simulink model "F550_CompareCA"  (R2024a)
settings: Solver=ode4  StartTime=0.0  StopTime=30  RelTol=1e-3
undefined symbols (not defined in the file or in its folder): r2d, SampleTime
libraries: slpidlib x21, simulink x9, simulink_extras x5
(part 1 of 3)
settings Model: Creator=UASG  LastModifiedBy=UASG

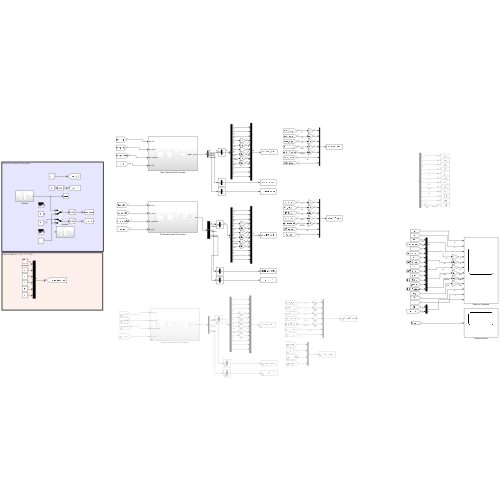
[thumbnail: Simulink's stored preview of the top-level diagram]
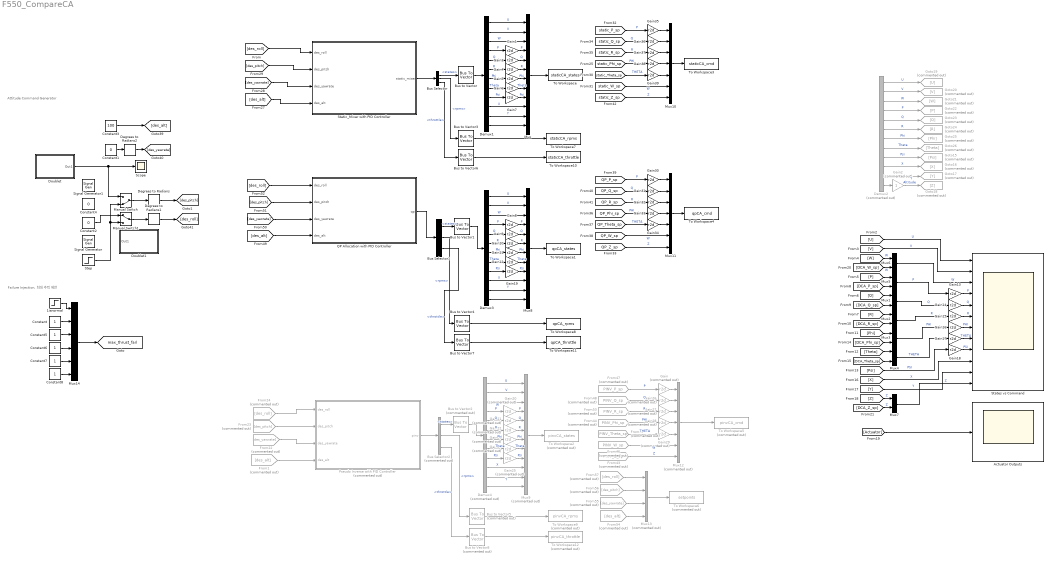
== system F550_CompareCA ==
  note: Failure Injection, 최대 추력 제한
  note: Attitude Command Generator
  1isnormal : Step  Time=10  Before=1  After=0.5
  Actuator Outputs : Scope
  Bus Selector : BusSelector  OutputSignals=states,rpms,throttle
  Bus Selector1 : BusSelector  OutputSignals=states,rpms,throttle
  Bus Selector2 : BusSelector  Commented=on  OutputSignals=states,rpms,throttle
  Bus to Vector{,1,3..4,6..7} (6 alike) : BusToVector
  Bus to Vector2 : BusToVector  Commented=on
  Bus to Vector5 : BusToVector  Commented=on
  Bus to Vector8 : BusToVector  Commented=on
  Constant{,5..8} (5 alike) : Constant
  Constant1 : Constant  Value=0
  Constant2 : Constant  Value=0
  Constant3 : Constant  Value=100
  Constant4 : Constant  Value=0
  Degrees to Radians : simulink_extras/Transformations/Degrees to Radians
  Degrees to Radians1 : simulink_extras/Transformations/Degrees to Radians
  Degrees to Radians2 : simulink_extras/Transformations/Degrees to Radians
  Demux1 : Demux  Outputs=12
  Demux2 : Demux  Commented=on  Outputs=12
  Demux3 : Demux  Outputs=12
  Demux4 : Demux  Commented=on  Outputs=12
  Doublet : Subsystem
  Doublet1 : Subsystem
  From1 : From  Commented=on  GotoTag=des_alt
  From22 : From  Commented=on  GotoTag=des_yawrate
  From23 : From  Commented=on  GotoTag=des_pitch
  From24 : From  Commented=on  GotoTag=des_roll
  From43 : From  Commented=on  GotoTag=PINV_Z_sp  TagVisibility=global
  From44 : From  Commented=on  GotoTag=PINV_Phi_sp  TagVisibility=global
  From45 : From  Commented=on  GotoTag=PINV_Theta_sp  TagVisibility=global
  From46 : From  Commented=on  GotoTag=PINV_W_sp  TagVisibility=global
  From47 : From  Commented=on  GotoTag=PINV_P_sp  TagVisibility=global
  From48 : From  Commented=on  GotoTag=PINV_Q_sp  TagVisibility=global
  From53 : From  Commented=on  GotoTag=PINV_R_sp  TagVisibility=global
  From54 : From  Commented=on  GotoTag=des_alt
  From55 : From  Commented=on  GotoTag=des_yawrate
  From56 : From  Commented=on  GotoTag=des_pitch
  From57 : From  Commented=on  GotoTag=des_roll
  Gain{,20..29} (11 alike) : Gain  Commented=on  Gain=r2d
  Gain{1,3..19,30..39} (28 alike) : Gain  Gain=r2d
  Gain2 : Gain  Commented=on
  Goto15 : Goto  Commented=on  GotoTag=Psi
  Goto16 : Goto  Commented=on  GotoTag=X
  Goto17 : Goto  Commented=on  GotoTag=Y
  Goto18 : Goto  Commented=on  GotoTag=Z
  Goto19 : Goto  Commented=on  GotoTag=U
  Goto20 : Goto  Commented=on  GotoTag=V
  Goto21 : Goto  Commented=on  GotoTag=W
  Goto22 : Goto  Commented=on  GotoTag=P
  Goto23 : Goto  Commented=on  GotoTag=Q
  Goto24 : Goto  Commented=on  GotoTag=R
  Goto25 : Goto  Commented=on  GotoTag=Phi
  Goto26 : Goto  Commented=on  GotoTag=Theta
  Manual Switch : ManualSwitch  CurrentSetting=0
  Manual Switch1 : ManualSwitch
  Mux : Mux  Inputs=12
  Mux{1..7} (7 alike) : Mux  Inputs=2
  Mux10 : Mux  Inputs=7
  Mux11 : Mux  Inputs=7
  Mux12 : Mux  Commented=on  Inputs=7
  Mux13 : Mux  Commented=on
  Mux14 : Mux  Inputs=6
  Mux8 : Mux  Inputs=12
  Mux9 : Mux  Commented=on  Inputs=12
  Pseudo Inverse with PID Controller : Subsystem  Commented=on
  QP Allocation with PID Controller : Subsystem
  Scope : Scope
  Signal Generator : SignalGenerator  Amplitude=4  Frequency=1/2
  Signal Generator1 : SignalGenerator  Amplitude=4  Frequency=1/2
  States vs Command : Scope  NumInputPorts=12
  Static_Mixer with PID Controller : Subsystem
  Step : Step  Time=5  After=10  SampleTime=0
  To Workspace : ToWorkspace  VariableName=staticCA_states  SampleTime=-1
  To Workspace1 : ToWorkspace  VariableName=qpCA_states  SampleTime=-1
  To Workspace10 : ToWorkspace  VariableName=staticCA_throttle  SampleTime=-1
      settings: Save2DSignal=2-D array (concatenate along first dimension)
  To Workspace11 : ToWorkspace  VariableName=qpCA_throttle  SampleTime=-1
      settings: Save2DSignal=2-D array (concatenate along first dimension)
  To Workspace12 : ToWorkspace  Commented=on  VariableName=pinvCA_throttle  SampleTime=-1
      settings: Save2DSignal=2-D array (concatenate along first dimension)
  To Workspace2 : ToWorkspace  Commented=on  VariableName=pinvCA_states  SampleTime=-1
  To Workspace3 : ToWorkspace  VariableName=staticCA_cmd  SampleTime=-1
  To Workspace4 : ToWorkspace  VariableName=qpCA_cmd  SampleTime=-1
  To Workspace5 : ToWorkspace  Commented=on  VariableName=pinvCA_cmd  SampleTime=-1
  To Workspace6 : ToWorkspace  Commented=on  VariableName=setpoints  SampleTime=-1
  To Workspace7 : ToWorkspace  VariableName=staticCA_rpms  SampleTime=-1
  To Workspace8 : ToWorkspace  VariableName=qpCA_rpms  SampleTime=-1
  To Workspace9 : ToWorkspace  Commented=on  VariableName=pinvCA_rpms  SampleTime=-1
  tag scope: max_thrust_fail=global
  wires:
  Constant2/1 -> Manual Switch1/1
  Degrees to Radians2/1 -> [des_yawrate]
  Degrees to Radians/1 -> [des_pitch]
  Degrees to Radians1/1 -> [des_roll]
  Manual Switch1/1 -> Degrees to Radians1/1
  Manual Switch/1 -> Degrees to Radians/1
  Constant1/1 -> Degrees to Radians2/1
  Constant3/1 -> [des_alt]
  Doublet/1(Out1) -> Manual Switch/1, Scope/1
  [DCA_Z_sp] -> Mux7/2  "Z"
  [Q] -> Mux1/1
  Gain18/1 -> States vs Command/9  "PSI"
  Gain15/1 -> States vs Command/6  "R"
  Gain17/1 -> States vs Command/8  "THETA"
  [DCA_W_sp] -> Mux6/2  "W"
  Gain16/1 -> States vs Command/7  "PHI"
  Gain13/1 -> States vs Command/4  "P"
  [DCA_Q_sp] -> Mux1/2
  [Phi] -> Mux3/1
  [DCA_Theta_sp] -> Mux4/2
  [Z] -> Mux7/1  "Z"
  [Actuator] -> Actuator Outputs/1
  [R] -> Mux2/1
  [Theta] -> Mux4/1
  [Psi] -> Gain18/1  "PSI"
  Mux4/1 -> Gain17/1  "THETA"
  Mux1/1 -> Gain14/1  "Q"
  Mux7/1 -> States vs Command/12  "Z"
  [X] -> States vs Command/10  "X"
  Mux3/1 -> Gain16/1  "PHI"
  Mux2/1 -> Gain15/1  "R"
  Mux6/1 -> States vs Command/3  "W"
  [W] -> Mux6/1  "W"
  Gain14/1 -> States vs Command/5  "Q"
  [DCA_Phi_sp] -> Mux3/2
  [V] -> States vs Command/2  "V"
  [U] -> States vs Command/1  "U"
  [P] -> Mux5/1
  [DCA_R_sp] -> Mux2/2
  Mux5/1 -> Gain13/1  "P"
  [Y] -> States vs Command/11  "Y"
  [DCA_P_sp] -> Mux5/2
  Gain2/1 -> Goto18/1  "Altitude"
  Demux2/12 -> Gain2/1
  Demux2/6 -> Goto24/1  "R"
  Demux2/9 -> Goto15/1  "Psi"
  Demux2/2 -> Goto20/1  "V"
  Demux2/5 -> Goto23/1  "Q"
  Demux2/4 -> Goto22/1  "P"
  Demux2/8 -> Goto26/1  "Theta"
  Demux2/3 -> Goto21/1  "W"
  Demux2/1 -> Goto19/1  "U"
  Demux2/11 -> Goto17/1  "Y"
  Demux2/10 -> Goto16/1  "X"
  Demux2/7 -> Goto25/1  "Phi"
  [des_roll] -> Static_Mixer with PID Controller/1(des_roll)
  [des_pitch] -> Static_Mixer with PID Controller/2(des_pitch)
  [des_yawrate] -> Static_Mixer with PID Controller/3(des_yawrate)
  [des_alt] -> Static_Mixer with PID Controller/4(des_alt)
  [des_roll] -> QP Allocation with PID Controller/1(des_roll)
  [des_pitch] -> QP Allocation with PID Controller/2(des_pitch)
  [des_yawrate] -> QP Allocation with PID Controller/3(des_yawrate)
  [des_alt] -> QP Allocation with PID Controller/4(des_alt)
  From24/1 -> Pseudo Inverse with PID Controller/1(des_roll)
  From23/1 -> Pseudo Inverse with PID Controller/2(des_pitch)
  From22/1 -> Pseudo Inverse with PID Controller/3(des_yawrate)
  From1/1 -> Pseudo Inverse with PID Controller/4(des_alt)
  Bus to Vector/1 -> Demux1/1
  Demux1/1 -> Mux/1  "U"
  Demux1/2 -> Mux/2  "V"
  Demux1/3 -> Mux/3  "W"
  Demux1/4 -> Gain1/1  "P"
  Gain1/1 -> Mux/4  "P"
  Demux1/5 -> Gain3/1  "Q"
  Gain3/1 -> Mux/5  "Q"
  Demux1/6 -> Gain4/1  "R"
  Demux1/7 -> Gain5/1  "Phi"
  Demux1/8 -> Gain6/1  "Theta"
  Demux1/9 -> Gain7/1  "Psi"
  Demux1/10 -> Mux/10  "X"
  Demux1/11 -> Mux/11  "Y"
  Demux1/12 -> Mux/12
  Gain7/1 -> Mux/9  "Psi"
  Gain6/1 -> Mux/8  "Theta"
  Gain5/1 -> Mux/7  "Phi"
  Gain4/1 -> Mux/6  "R"
  Mux/1 -> To Workspace/1
  Bus to Vector1/1 -> Demux3/1
  Gain10/1 -> Mux8/6  "R"
  Gain19/1 -> Mux8/9  "Psi"
  Gain11/1 -> Mux8/7  "Phi"
  Gain12/1 -> Mux8/8  "Theta"
  Demux3/8 -> Gain12/1  "Theta"
  Demux3/10 -> Mux8/10  "X"
  Gain9/1 -> Mux8/5  "Q"
  Demux3/3 -> Mux8/3  "W"
  Gain8/1 -> Mux8/4  "P"
  Demux3/12 -> Mux8/12
  Demux3/2 -> Mux8/2  "V"
  Demux3/11 -> Mux8/11  "Y"
  Demux3/4 -> Gain8/1  "P"
  Demux3/9 -> Gain19/1  "Psi"
  Mux8/1 -> To Workspace1/1
  Demux3/5 -> Gain9/1  "Q"
  Demux3/7 -> Gain11/1  "Phi"
  Demux3/6 -> Gain10/1  "R"
  Demux3/1 -> Mux8/1  "U"
  Bus to Vector2/1 -> Demux4/1
  Gain22/1 -> Mux9/6  "R"
  Gain25/1 -> Mux9/9  "Psi"
  Gain23/1 -> Mux9/7  "Phi"
  Gain24/1 -> Mux9/8  "Theta"
  Demux4/8 -> Gain24/1  "Theta"
  Demux4/10 -> Mux9/10  "X"
  Gain21/1 -> Mux9/5  "Q"
  Demux4/3 -> Mux9/3  "W"
  Gain20/1 -> Mux9/4  "P"
  Demux4/12 -> Mux9/12
  Demux4/2 -> Mux9/2  "V"
  Demux4/11 -> Mux9/11  "Y"
  Demux4/4 -> Gain20/1  "P"
  Demux4/9 -> Gain25/1  "Psi"
  Mux9/1 -> To Workspace2/1
  Demux4/5 -> Gain21/1  "Q"
  Demux4/7 -> Gain23/1  "Phi"
  Demux4/6 -> Gain22/1  "R"
  Demux4/1 -> Mux9/1  "U"
  [static_P_sp] -> Gain35/1  "P"
  [static_Q_sp] -> Gain36/1  "Q"
  [static_R_sp] -> Gain37/1  "R"
  [static_Phi_sp] -> Gain38/1  "PHI"
  [static_Theta_sp] -> Gain39/1  "THETA"
  [static_W_sp] -> Mux10/6  "W"
  Mux10/1 -> To Workspace3/1
  [QP_P_sp] -> Gain30/1  "P"
  [QP_R_sp] -> Gain32/1  "R"
  [QP_Theta_sp] -> Gain34/1  "THETA"
  [QP_Phi_sp] -> Gain33/1  "PHI"
  Mux11/1 -> To Workspace4/1
  [QP_W_sp] -> Mux11/6  "W"
  [QP_Q_sp] -> Gain31/1  "Q"
  [static_Z_sp] -> Mux10/7  "Z"
  [QP_Z_sp] -> Mux11/7  "Z"
  From46/1 -> Mux12/6  "W"
  From47/1 -> Gain/1  "P"
  From44/1 -> Gain28/1  "PHI"
  From48/1 -> Gain26/1  "Q"
  From43/1 -> Mux12/7  "Z"
  From53/1 -> Gain27/1  "R"
  From45/1 -> Gain29/1  "THETA"
  From57/1 -> Mux13/1
  From56/1 -> Mux13/2
  From55/1 -> Mux13/3
  From54/1 -> Mux13/4
  Mux13/1 -> To Workspace6/1
  Mux12/1 -> To Workspace5/1
  Gain/1 -> Mux12/1
  Gain26/1 -> Mux12/2
  Gain27/1 -> Mux12/3
  Gain28/1 -> Mux12/4
  Gain29/1 -> Mux12/5
  Gain30/1 -> Mux11/1
  Gain31/1 -> Mux11/2
  Gain32/1 -> Mux11/3
  Gain33/1 -> Mux11/4
  Gain34/1 -> Mux11/5
  Gain35/1 -> Mux10/1
  Gain36/1 -> Mux10/2
  Gain37/1 -> Mux10/3
  Gain38/1 -> Mux10/4
  Gain39/1 -> Mux10/5
  Static_Mixer with PID Controller/1(static_mixer) -> Bus Selector/1
  Bus Selector/1 -> Bus to Vector/1  "<states>"
  Bus Selector/2 -> Bus to Vector3/1  "<rpms>"
  Bus to Vector3/1 -> To Workspace7/1
  QP Allocation with PID Controller/1(qp) -> Bus Selector1/1
  Bus Selector1/1 -> Bus to Vector1/1  "<states>"
  Bus Selector1/2 -> Bus to Vector4/1  "<rpms>"
  Bus to Vector4/1 -> To Workspace8/1
  Pseudo Inverse with PID Controller/1(pinv) -> Bus Selector2/1
  Bus Selector2/1 -> Bus to Vector2/1  "<states>"
  Bus Selector2/2 -> Bus to Vector5/1  "<rpms>"
  Bus to Vector5/1 -> To Workspace9/1
  Bus Selector/3 -> Bus to Vector6/1  "<throttle>"
  Bus to Vector6/1 -> To Workspace10/1
  Bus to Vector7/1 -> To Workspace11/1
  Bus to Vector8/1 -> To Workspace12/1
  Bus Selector1/3 -> Bus to Vector7/1  "<throttle>"
  Bus Selector2/3 -> Bus to Vector8/1  "<throttle>"
  Step/1 -> Manual Switch/2, Manual Switch1/2
  1isnormal/1 -> Mux14/1
  Constant/1 -> Mux14/2
  Constant5/1 -> Mux14/3
  Constant6/1 -> Mux14/4
  Constant7/1 -> Mux14/5
  Constant8/1 -> Mux14/6
  Mux14/1 -> [max_thrust_fail]

== system F550_CompareCA/Doublet ==
  Add : Sum  Inputs=+++
  Step : Step  Time=10  After=8  SampleTime=0
  Step1 : Step  Time=15  After=-16  SampleTime=0
  Step2 : Step  Time=20  After=8  SampleTime=0
  Out1 : Outport
  wires:
  Step/1 -> Add/1
  Step1/1 -> Add/2
  Add/1 -> Out1/1
  Step2/1 -> Add/3

== system F550_CompareCA/Doublet1 ==
  Add : Sum  Inputs=+++
  Step : Step  Time=10  After=10  SampleTime=0
  Step1 : Step  Time=15  After=-20  SampleTime=0
  Step2 : Step  Time=20  After=10  SampleTime=0
  Out1 : Outport
  wires:
  Step/1 -> Add/1
  Step1/1 -> Add/2
  Add/1 -> Out1/1
  Step2/1 -> Add/3

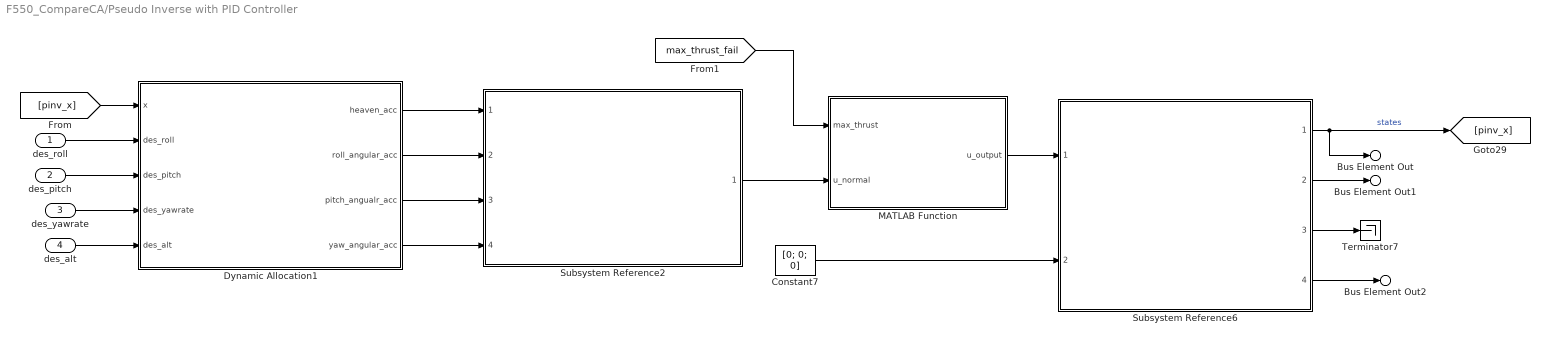
== system F550_CompareCA/Pseudo Inverse with PID Controller ==
  des_roll : Inport
  des_pitch : Inport  Port=2
  des_yawrate : Inport  Port=3
  des_alt : Inport  Port=4
  Constant7 : Constant  Value=[0; 0; 0]
  Dynamic Allocation1 : Subsystem
  MATLAB Function : MATLAB Function  TreatAsAtomicUnit=on
  Subsystem Reference2 : Subsystem  ReferencedSubsystem=F550_PseudoInv_ControlAllocation
  Subsystem Reference6 : Subsystem  ReferencedSubsystem=F550_Dynamics_sub_ver2023b
  Terminator7 : Terminator
  Bus Element Out : Outport  PortName=pinv  Element=states
  Bus Element Out1 : Outport  PortName=pinv  Element=rpms
  Bus Element Out2 : Outport  PortName=pinv  Element=throttle
  wires:
  Dynamic Allocation1/3(pitch_angualr_acc) -> Subsystem Reference2/3
  Dynamic Allocation1/1(heaven_acc) -> Subsystem Reference2/1
  Subsystem Reference6/1 -> Bus Element Out/1, [pinv_x]  "states"
  Dynamic Allocation1/4(yaw_angular_acc) -> Subsystem Reference2/4
  Subsystem Reference6/2 -> Bus Element Out1/1
  Dynamic Allocation1/2(roll_angular_acc) -> Subsystem Reference2/2
  Constant7/1 -> Subsystem Reference6/2
  des_yawrate/1 -> Dynamic Allocation1/4(des_yawrate)
  Subsystem Reference6/3 -> Terminator7/1
  des_roll/1 -> Dynamic Allocation1/2(des_roll)
  des_pitch/1 -> Dynamic Allocation1/3(des_pitch)
  des_alt/1 -> Dynamic Allocation1/5(des_alt)
  [pinv_x] -> Dynamic Allocation1/1(x)
  Subsystem Reference6/4 -> Bus Element Out2/1
  [max_thrust_fail] -> MATLAB Function/1(max_thrust)
  Subsystem Reference2/1 -> MATLAB Function/2(u_normal)
  MATLAB Function/1(u_output) -> Subsystem Reference6/1

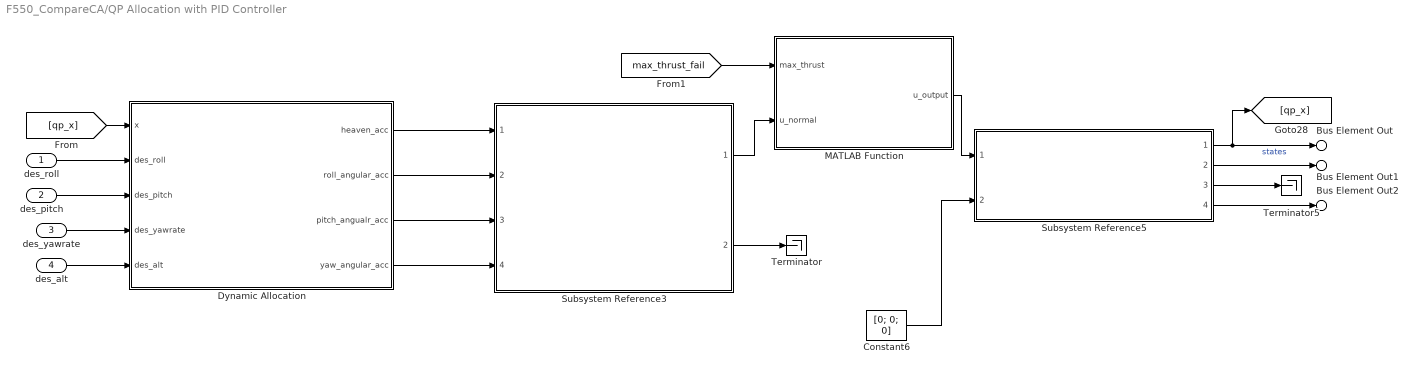
== system F550_CompareCA/QP Allocation with PID Controller ==
  des_roll : Inport
  des_pitch : Inport  Port=2
  des_yawrate : Inport  Port=3
  des_alt : Inport  Port=4
  Constant6 : Constant  Value=[0; 0; 0]
  Dynamic Allocation : Subsystem
  MATLAB Function : MATLAB Function  TreatAsAtomicUnit=on
  Subsystem Reference3 : Subsystem  ReferencedSubsystem=F550_Dynamic_CA
  Subsystem Reference5 : Subsystem  ReferencedSubsystem=F550_Dynamics_sub_ver2023b
  Terminator : Terminator
  Terminator5 : Terminator
  Bus Element Out : Outport  PortName=qp  Element=states
  Bus Element Out1 : Outport  PortName=qp  Element=rpms
  Bus Element Out2 : Outport  PortName=qp  Element=throttle
  wires:
  Subsystem Reference5/1 -> Bus Element Out/1, [qp_x]  "states"
  Dynamic Allocation/4(yaw_angular_acc) -> Subsystem Reference3/4
  Constant6/1 -> Subsystem Reference5/2
  Dynamic Allocation/3(pitch_angualr_acc) -> Subsystem Reference3/3
  Subsystem Reference5/3 -> Terminator5/1
  Dynamic Allocation/1(heaven_acc) -> Subsystem Reference3/1
  Dynamic Allocation/2(roll_angular_acc) -> Subsystem Reference3/2
  Subsystem Reference5/2 -> Bus Element Out1/1
  des_yawrate/1 -> Dynamic Allocation/4(des_yawrate)
  des_pitch/1 -> Dynamic Allocation/3(des_pitch)
  des_alt/1 -> Dynamic Allocation/5(des_alt)
  des_roll/1 -> Dynamic Allocation/2(des_roll)
  Subsystem Reference3/2 -> Terminator/1
  [qp_x] -> Dynamic Allocation/1(x)
  Subsystem Reference5/4 -> Bus Element Out2/1
  [max_thrust_fail] -> MATLAB Function/1(max_thrust)
  Subsystem Reference3/1 -> MATLAB Function/2(u_normal)
  MATLAB Function/1(u_output) -> Subsystem Reference5/1

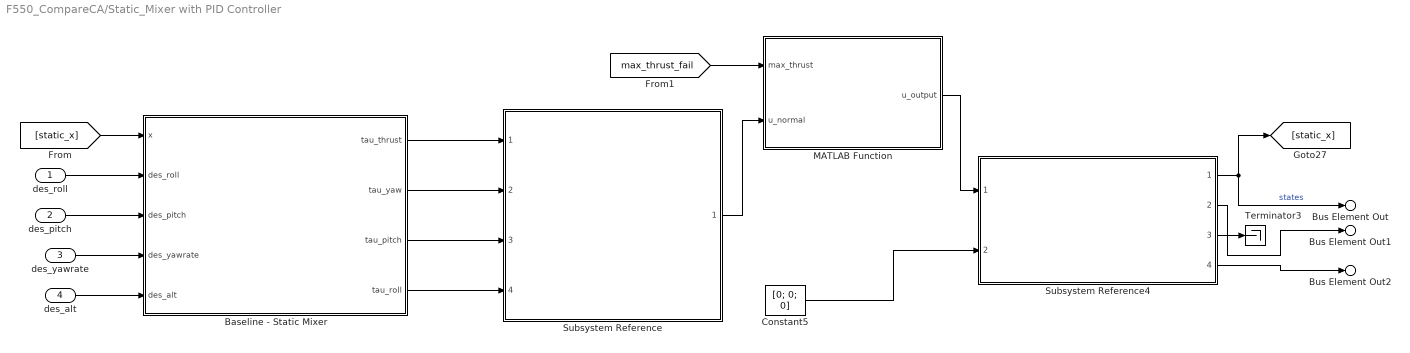
== system F550_CompareCA/Static_Mixer with PID Controller ==
  des_roll : Inport
  des_pitch : Inport  Port=2
  des_yawrate : Inport  Port=3
  des_alt : Inport  Port=4
  Baseline - Static Mixer : Subsystem
  Constant5 : Constant  Value=[0; 0; 0]
  MATLAB Function : MATLAB Function  TreatAsAtomicUnit=on
  Subsystem Reference : Subsystem  ReferencedSubsystem=F550_ControlAllocation_sub_ver2023b
  Subsystem Reference4 : Subsystem  ReferencedSubsystem=F550_Dynamics_sub_ver2023b
  Terminator3 : Terminator
  Bus Element Out : Outport  PortName=static_mixer  Element=states
  Bus Element Out1 : Outport  PortName=static_mixer  Element=rpms
  Bus Element Out2 : Outport  PortName=static_mixer  Element=throttle
  wires:
  Baseline - Static Mixer/4(tau_roll) -> Subsystem Reference/4
  Baseline - Static Mixer/2(tau_yaw) -> Subsystem Reference/2
  Baseline - Static Mixer/1(tau_thrust) -> Subsystem Reference/1
  Subsystem Reference4/1 -> Bus Element Out/1, [static_x]  "states"
  Baseline - Static Mixer/3(tau_pitch) -> Subsystem Reference/3
  Subsystem Reference4/3 -> Terminator3/1
  des_yawrate/1 -> Baseline - Static Mixer/4(des_yawrate)
  Constant5/1 -> Subsystem Reference4/2
  Subsystem Reference4/2 -> Bus Element Out1/1
  des_pitch/1 -> Baseline - Static Mixer/3(des_pitch)
  des_alt/1 -> Baseline - Static Mixer/5(des_alt)
  des_roll/1 -> Baseline - Static Mixer/2(des_roll)
  [static_x] -> Baseline - Static Mixer/1(x)
  Subsystem Reference4/4 -> Bus Element Out2/1
  Subsystem Reference/1 -> MATLAB Function/2(u_normal)
  MATLAB Function/1(u_output) -> Subsystem Reference4/1
  [max_thrust_fail] -> MATLAB Function/1(max_thrust)

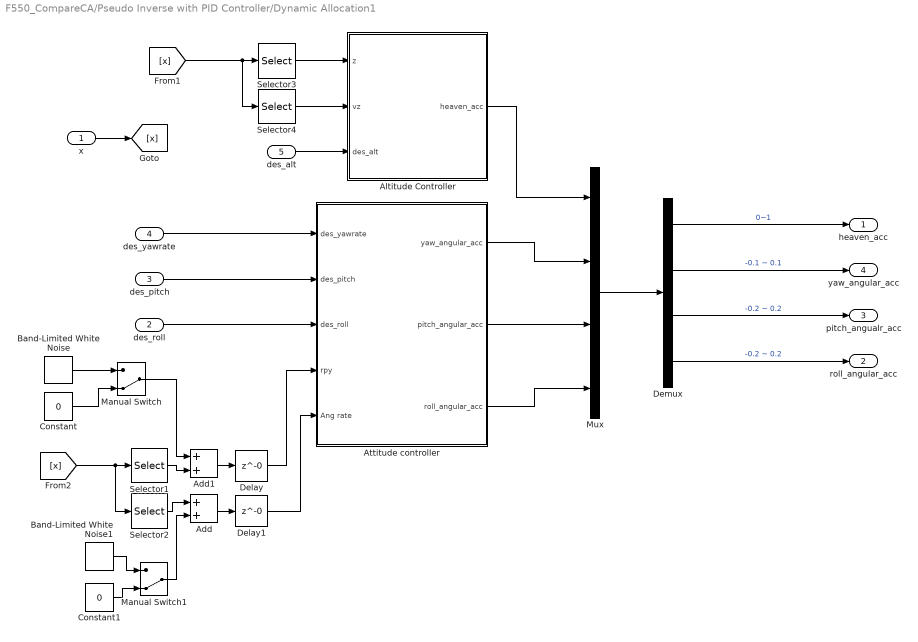
== system F550_CompareCA/Pseudo Inverse with PID Controller/Dynamic Allocation1 ==
  x : Inport
  des_roll : Inport  Port=2
  des_pitch : Inport  Port=3
  des_yawrate : Inport  Port=4
  des_alt : Inport  Port=5
  Add : Sum
  Add1 : Sum
  Altitude Controller : Subsystem
  Attitude controller : Subsystem
  Band-Limited White Noise : simulink/Sources/Band-Limited White Noise  Cov=[1e-5]  Ts=SampleTime  seed=[23341]
  Band-Limited White Noise1 : simulink/Sources/Band-Limited White Noise  Cov=[1e-6]  Ts=SampleTime  seed=[23341]
  Constant : Constant  Value=0
  Constant1 : Constant  Value=0
  Delay : Delay  DelayLength=0
  Delay1 : Delay  DelayLength=0
  Demux : Demux
  Manual Switch : ManualSwitch  CurrentSetting=0
  Manual Switch1 : ManualSwitch  CurrentSetting=0
  Mux : Mux
  Selector1 : Selector  InputPortWidth=12  IndexOptions=Index vector (dialog)  Indices=[7 8 9]  OutputSizes=1
  Selector2 : Selector  InputPortWidth=12  IndexOptions=Index vector (dialog)  Indices=[4 5 6]  OutputSizes=1
  Selector3 : Selector  InputPortWidth=12  IndexOptions=Index vector (dialog)  Indices=[12]  OutputSizes=1
  Selector4 : Selector  InputPortWidth=12  IndexOptions=Index vector (dialog)  Indices=[3]  OutputSizes=1
  heaven_acc : Outport
  roll_angular_acc : Outport  Port=2
  pitch_angualr_acc : Outport  Port=3
  yaw_angular_acc : Outport  Port=4
  wires:
  Add1/1 -> Delay/1
  Add/1 -> Delay1/1
  Selector2/1 -> Add/1
  Attitude controller/2(pitch_angular_acc) -> Mux/3
  Selector3/1 -> Altitude Controller/1(z)
  Selector4/1 -> Altitude Controller/2(vz)
  Attitude controller/3(roll_angular_acc) -> Mux/4
  Attitude controller/1(yaw_angular_acc) -> Mux/2
  Altitude Controller/1(heaven_acc) -> Mux/1
  Demux/2 -> yaw_angular_acc/1  "-0.1 ~ 0.1"
  Mux/1 -> Demux/1
  Demux/1 -> heaven_acc/1  "0~1"
  Demux/3 -> pitch_angualr_acc/1  "-0.2 ~ 0.2"
  Demux/4 -> roll_angular_acc/1  "-0.2 ~ 0.2"
  Delay/1 -> Attitude controller/4(rpy)
  [x] -> Selector4/1, Selector3/1
  Delay1/1 -> Attitude controller/5(Ang rate)
  [x] -> Selector2/1, Selector1/1
  x/1 -> [x]
  des_roll/1 -> Attitude controller/3(des_roll)
  des_pitch/1 -> Attitude controller/2(des_pitch)
  des_yawrate/1 -> Attitude controller/1(des_yawrate)
  des_alt/1 -> Altitude Controller/3(des_alt)
  Band-Limited White Noise/1 -> Manual Switch/1
  Selector1/1 -> Add1/2
  Manual Switch/1 -> Add1/1
  Constant/1 -> Manual Switch/2
  Band-Limited White Noise1/1 -> Manual Switch1/1
  Constant1/1 -> Manual Switch1/2
  Manual Switch1/1 -> Add/2

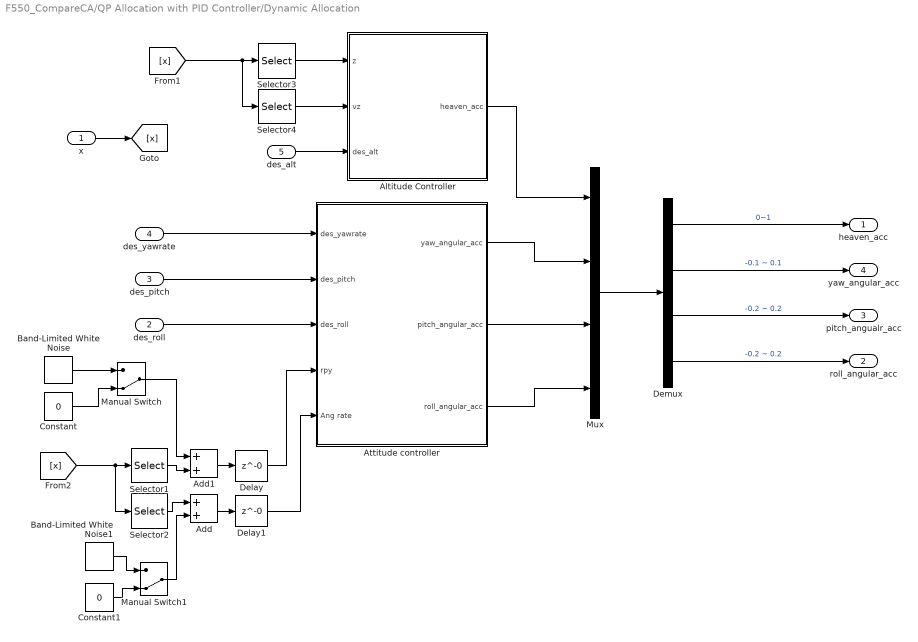
== system F550_CompareCA/QP Allocation with PID Controller/Dynamic Allocation ==
  x : Inport
  des_roll : Inport  Port=2
  des_pitch : Inport  Port=3
  des_yawrate : Inport  Port=4
  des_alt : Inport  Port=5
  Add : Sum
  Add1 : Sum
  Altitude Controller : Subsystem
  Attitude controller : Subsystem
  Band-Limited White Noise : simulink/Sources/Band-Limited White Noise  Cov=[1e-5]  Ts=SampleTime  seed=[23341]
  Band-Limited White Noise1 : simulink/Sources/Band-Limited White Noise  Cov=[1e-6]  Ts=SampleTime  seed=[23341]
  Constant : Constant  Value=0
  Constant1 : Constant  Value=0
  Delay : Delay  DelayLength=0
  Delay1 : Delay  DelayLength=0
  Demux : Demux
  Manual Switch : ManualSwitch  CurrentSetting=0
  Manual Switch1 : ManualSwitch  CurrentSetting=0
  Mux : Mux
  Selector1 : Selector  InputPortWidth=12  IndexOptions=Index vector (dialog)  Indices=[7 8 9]  OutputSizes=1
  Selector2 : Selector  InputPortWidth=12  IndexOptions=Index vector (dialog)  Indices=[4 5 6]  OutputSizes=1
  Selector3 : Selector  InputPortWidth=12  IndexOptions=Index vector (dialog)  Indices=[12]  OutputSizes=1
  Selector4 : Selector  InputPortWidth=12  IndexOptions=Index vector (dialog)  Indices=[3]  OutputSizes=1
  heaven_acc : Outport
  roll_angular_acc : Outport  Port=2
  pitch_angualr_acc : Outport  Port=3
  yaw_angular_acc : Outport  Port=4
  wires:
  Add1/1 -> Delay/1
  Add/1 -> Delay1/1
  Selector2/1 -> Add/1
  Attitude controller/2(pitch_angular_acc) -> Mux/3
  Selector3/1 -> Altitude Controller/1(z)
  Selector4/1 -> Altitude Controller/2(vz)
  Attitude controller/3(roll_angular_acc) -> Mux/4
  Attitude controller/1(yaw_angular_acc) -> Mux/2
  Altitude Controller/1(heaven_acc) -> Mux/1
  Demux/2 -> yaw_angular_acc/1  "-0.1 ~ 0.1"
  Mux/1 -> Demux/1
  Demux/1 -> heaven_acc/1  "0~1"
  Demux/3 -> pitch_angualr_acc/1  "-0.2 ~ 0.2"
  Demux/4 -> roll_angular_acc/1  "-0.2 ~ 0.2"
  Delay/1 -> Attitude controller/4(rpy)
  [x] -> Selector4/1, Selector3/1
  Delay1/1 -> Attitude controller/5(Ang rate)
  [x] -> Selector2/1, Selector1/1
  x/1 -> [x]
  des_roll/1 -> Attitude controller/3(des_roll)
  des_pitch/1 -> Attitude controller/2(des_pitch)
  des_yawrate/1 -> Attitude controller/1(des_yawrate)
  des_alt/1 -> Altitude Controller/3(des_alt)
  Band-Limited White Noise/1 -> Manual Switch/1
  Selector1/1 -> Add1/2
  Manual Switch/1 -> Add1/1
  Constant/1 -> Manual Switch/2
  Band-Limited White Noise1/1 -> Manual Switch1/1
  Constant1/1 -> Manual Switch1/2
  Manual Switch1/1 -> Add/2

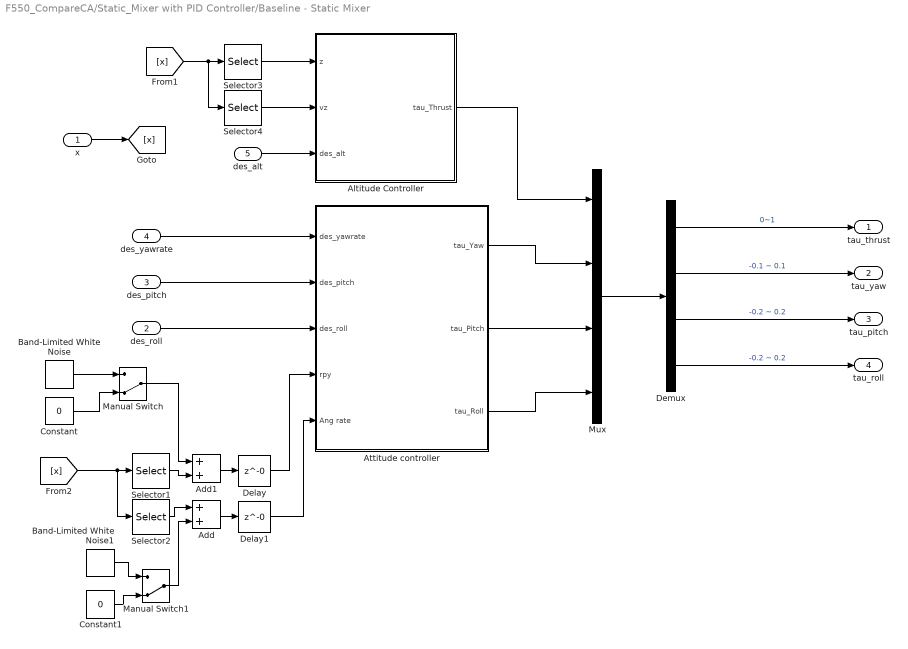
== system F550_CompareCA/Static_Mixer with PID Controller/Baseline - Static Mixer ==
  x : Inport
  des_roll : Inport  Port=2
  des_pitch : Inport  Port=3
  des_yawrate : Inport  Port=4
  des_alt : Inport  Port=5
  Add : Sum
  Add1 : Sum
  Altitude Controller : Subsystem
  Attitude controller : Subsystem
  Band-Limited White Noise : simulink/Sources/Band-Limited White Noise  Cov=[1e-5]  Ts=SampleTime  seed=[23341]
  Band-Limited White Noise1 : simulink/Sources/Band-Limited White Noise  Cov=[1e-6]  Ts=SampleTime  seed=[23341]
  Constant : Constant  Value=0
  Constant1 : Constant  Value=0
  Delay : Delay  DelayLength=0
  Delay1 : Delay  DelayLength=0
  Demux : Demux
  Manual Switch : ManualSwitch  CurrentSetting=0
  Manual Switch1 : ManualSwitch  CurrentSetting=0
  Mux : Mux
  Selector1 : Selector  InputPortWidth=12  IndexOptions=Index vector (dialog)  Indices=[7 8 9]  OutputSizes=1
  Selector2 : Selector  InputPortWidth=12  IndexOptions=Index vector (dialog)  Indices=[4 5 6]  OutputSizes=1
  Selector3 : Selector  InputPortWidth=12  IndexOptions=Index vector (dialog)  Indices=[12]  OutputSizes=1
  Selector4 : Selector  InputPortWidth=12  IndexOptions=Index vector (dialog)  Indices=[3]  OutputSizes=1
  tau_thrust : Outport
  tau_yaw : Outport  Port=2
  tau_pitch : Outport  Port=3
  tau_roll : Outport  Port=4
  wires:
  Attitude controller/2(tau_Pitch) -> Mux/3
  Selector3/1 -> Altitude Controller/1(z)
  Selector4/1 -> Altitude Controller/2(vz)
  Attitude controller/3(tau_Roll) -> Mux/4
  Attitude controller/1(tau_Yaw) -> Mux/2
  Altitude Controller/1(tau_Thrust) -> Mux/1
  Demux/2 -> tau_yaw/1  "-0.1 ~ 0.1"
  Mux/1 -> Demux/1
  Demux/1 -> tau_thrust/1  "0~1"
  Demux/3 -> tau_pitch/1  "-0.2 ~ 0.2"
  Demux/4 -> tau_roll/1  "-0.2 ~ 0.2"
  [x] -> Selector4/1, Selector3/1
  x/1 -> [x]
  des_roll/1 -> Attitude controller/3(des_roll)
  des_pitch/1 -> Attitude controller/2(des_pitch)
  des_yawrate/1 -> Attitude controller/1(des_yawrate)
  des_alt/1 -> Altitude Controller/3(des_alt)
  Manual Switch/1 -> Add1/1
  Constant1/1 -> Manual Switch1/2
  Band-Limited White Noise1/1 -> Manual Switch1/1
  Band-Limited White Noise/1 -> Manual Switch/1
  Manual Switch1/1 -> Add/2
  Constant/1 -> Manual Switch/2
  Selector1/1 -> Add1/2
  Delay1/1 -> Attitude controller/5(Ang rate)
  [x] -> Selector2/1, Selector1/1
  Selector2/1 -> Add/1
  Delay/1 -> Attitude controller/4(rpy)
  Add1/1 -> Delay/1
  Add/1 -> Delay1/1

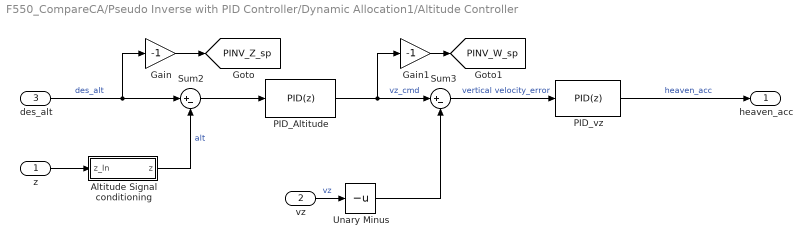
== system F550_CompareCA/Pseudo Inverse with PID Controller/Dynamic Allocation1/Altitude Controller ==
  z : Inport
  vz : Inport  Port=2
  des_alt : Inport  Port=3
  Altitude Signal conditioning : Subsystem
  Gain : Gain  Gain=-1
  Gain1 : Gain  Gain=-1
  PID_Altitude : slpidlib/PID Controller  Controller=PID  Form=Parallel  TimeDomain=Discrete-time  UseExternalTs=off  SampleTime=-1  IntegratorMethod=Backward Euler  FilterMethod=Forward Euler  ControllerParametersSource=internal  P=1  I=0  UseKiTs=off  D=0  UseExternalDerivativeSource=off  N=10  UseFilter=on  TunerSelectOption=Transfer Function Based (PID Tuner App)  InitialConditionSource=internal  InitialConditionForIntegrator=0  InitialConditionForFilter=0  DifferentiatorICPrevScaledInput=0  ExternalReset=none  TrackingMode=off  Kt=1  LimitOutput=on  SatLimitsSource=internal  UpperSaturationLimit=2  LowerSaturationLimit=-2  LinearizeAsGain=off  AntiWindupMode=clamping  Kb=1  LimitIntegrator=off  UpperIntegratorSaturationLimit=inf  LowerIntegratorSaturationLimit=-inf  POutMin=[]  POutMax=[]  IOutMin=[]  IOutMax=[]  DOutMin=[]  DOutMax=[]  NOutMin=[]  NOutMax=[]  SumOutMin=[]  SumOutMax=[]  SaturationOutMin=[]  SaturationOutMax=[]  PParamMin=[]  PParamMax=[]  IParamMin=[]  IParamMax=[]  DParamMin=[]  DParamMax=[]  NParamMin=[]  NParamMax=[]  KbParamMin=[]  KbParamMax=[]  KtParamMin=[]  KtParamMax=[]  KbOutMin=[]  KbOutMax=[]  KtOutMin=[]  KtOutMax=[]  IntegratorOutMin=[]  IntegratorOutMax=[]  FilterOutMin=[]  FilterOutMax=[]  SumI1OutMin=[]  SumI1OutMax=[]  SumI2OutMin=[]  SumI2OutMax=[]  SumI3OutMin=[]  SumI3OutMax=[]  SumI4OutMin=[]  SumI4OutMax=[]  SumDOutMin=[]  SumDOutMax=[]  DifferentiatorOutMin=[]  DifferentiatorOutMax=[]  FilterDiffOutCoefMin=[]  FilterDiffOutCoefMax=[]  ReciprocalOutMin=[]  ReciprocalOutMax=[]  SumDenOutMin=[]  SumDenOutMax=[]  SumNumOutMin=[]  SumNumOutMax=[]  DivideOutMin=[]  DivideOutMax=[]  UdiffTsProdOutMin=[]  UdiffTsProdOutMax=[]  NTsProdOutMin=[]  NTsProdOutMax=[]  UintegralTsProdOutMin=[]  UintegralTsProdOutMax=[]  UngainTsProdOutMin=[]  UngainTsProdOutMax=[]  ClampingZeroOutDataTypeStr=Inherit: Inherit via back propagation  ClampingZeroOutMin=[]  ClampingZeroOutMax=[]  FilterDenConstantOutDataTypeStr=Inherit: Inherit via back propagation  FilterDenConstantOutMin=[]  FilterDenConstantOutMax=[]  PCopyOutDataTypeStr=Inherit: Inherit via back propagation  PCopyOutMin=[]  PCopyOutMax=[]  NCopyOutDataTypeStr=Inherit: Inherit via back propagation  NCopyOutMin=[]  NCopyOutMax=[]  IntegratorContinuousStateAttributes=''  IntegratorStateMustResolveToSignalObject=off  IntegratorRTWStateStorageClass=Auto  FilterContinuousStateAttributes=''  FilterStateMustResolveToSignalObject=off  FilterRTWStateStorageClass=Auto  ParallelPVariant=InternalParameters  IdealPVariant=Disabled  IVariant=InternalParameters  DVariant=InternalParameters  IntegratorVariant=Discrete  SatVariant=Enabled  AWVariant=DiscClampingParallel  PCopyVariant=Disabled  TRVariant=Disabled  FdbkBlocksVariant=Feedback  IdealPFdbkVariant=Passthrough  SatFdbkVariant=Passthrough  DerivativeFilterVariant=ForwardEulerFilter  NVariant=InternalParameters  NCopyVariant=Disabled  FilterICVariant=InternalICsFilter  IntegratorICVariant=InternalICs  ExternalResetVariant=Disabled  TRSumVariant=Passthrough  SumFdbkVariant=Enabled  SumVariant=Sum_PID  TsampFilterVariant=InternalTs  TsampNgainVariant=Passthrough  TsampIntegralVariant=Disabled_SignalSpec  ExternalSaturationOutDataTypeStr=Inherit: Same as second input  DerivativeSourceVariant=ErrorSignal
  PID_vz : slpidlib/PID Controller  Controller=PID  Form=Parallel  TimeDomain=Discrete-time  UseExternalTs=off  SampleTime=-1  IntegratorMethod=Backward Euler  FilterMethod=Forward Euler  ControllerParametersSource=internal  P=4  I=2  UseKiTs=off  D=0  UseExternalDerivativeSource=off  N=10  UseFilter=on  TunerSelectOption=Transfer Function Based (PID Tuner App)  InitialConditionSource=internal  InitialConditionForIntegrator=0  InitialConditionForFilter=0  DifferentiatorICPrevScaledInput=0  ExternalReset=none  TrackingMode=off  Kt=1  LimitOutput=off  SatLimitsSource=internal  UpperSaturationLimit=1  LowerSaturationLimit=0  LinearizeAsGain=off  AntiWindupMode=clamping  Kb=1  LimitIntegrator=off  UpperIntegratorSaturationLimit=inf  LowerIntegratorSaturationLimit=-inf  POutMin=[]  POutMax=[]  IOutMin=[]  IOutMax=[]  DOutMin=[]  DOutMax=[]  NOutMin=[]  NOutMax=[]  SumOutMin=[]  SumOutMax=[]  SaturationOutMin=[]  SaturationOutMax=[]  PParamMin=[]  PParamMax=[]  IParamMin=[]  IParamMax=[]  DParamMin=[]  DParamMax=[]  NParamMin=[]  NParamMax=[]  KbParamMin=[]  KbParamMax=[]  KtParamMin=[]  KtParamMax=[]  KbOutMin=[]  KbOutMax=[]  KtOutMin=[]  KtOutMax=[]  IntegratorOutMin=[]  IntegratorOutMax=[]  FilterOutMin=[]  FilterOutMax=[]  SumI1OutMin=[]  SumI1OutMax=[]  SumI2OutMin=[]  SumI2OutMax=[]  SumI3OutMin=[]  SumI3OutMax=[]  SumI4OutMin=[]  SumI4OutMax=[]  SumDOutMin=[]  SumDOutMax=[]  DifferentiatorOutMin=[]  DifferentiatorOutMax=[]  FilterDiffOutCoefMin=[]  FilterDiffOutCoefMax=[]  ReciprocalOutMin=[]  ReciprocalOutMax=[]  SumDenOutMin=[]  SumDenOutMax=[]  SumNumOutMin=[]  SumNumOutMax=[]  DivideOutMin=[]  DivideOutMax=[]  UdiffTsProdOutMin=[]  UdiffTsProdOutMax=[]  NTsProdOutMin=[]  NTsProdOutMax=[]  UintegralTsProdOutMin=[]  UintegralTsProdOutMax=[]  UngainTsProdOutMin=[]  UngainTsProdOutMax=[]  ClampingZeroOutDataTypeStr=Inherit: Inherit via back propagation  ClampingZeroOutMin=[]  ClampingZeroOutMax=[]  FilterDenConstantOutDataTypeStr=Inherit: Inherit via back propagation  FilterDenConstantOutMin=[]  FilterDenConstantOutMax=[]  PCopyOutDataTypeStr=Inherit: Inherit via back propagation  PCopyOutMin=[]  PCopyOutMax=[]  NCopyOutDataTypeStr=Inherit: Inherit via back propagation  NCopyOutMin=[]  NCopyOutMax=[]  IntegratorContinuousStateAttributes=''  IntegratorStateMustResolveToSignalObject=off  IntegratorRTWStateStorageClass=Auto  FilterContinuousStateAttributes=''  FilterStateMustResolveToSignalObject=off  FilterRTWStateStorageClass=Auto  ParallelPVariant=InternalParameters  IdealPVariant=Disabled  IVariant=InternalParameters  DVariant=InternalParameters  IntegratorVariant=Discrete  SatVariant=Disabled  AWVariant=Passthrough  PCopyVariant=Disabled  TRVariant=Disabled  FdbkBlocksVariant=Forward  IdealPFdbkVariant=Disabled  SatFdbkVariant=Disabled  DerivativeFilterVariant=ForwardEulerFilter  NVariant=InternalParameters  NCopyVariant=Disabled  FilterICVariant=InternalICsFilter  IntegratorICVariant=InternalICs  ExternalResetVariant=Disabled  TRSumVariant=Passthrough  SumFdbkVariant=Disabled  SumVariant=Sum_PID  TsampFilterVariant=InternalTs  TsampNgainVariant=Passthrough  TsampIntegralVariant=Disabled_SignalSpec  ExternalSaturationOutDataTypeStr=Inherit: Same as second input  DerivativeSourceVariant=ErrorSignal
  Sum2 : Sum  Inputs=|+-
  Sum3 : Sum  Inputs=|+-
  Unary Minus : UnaryMinus
  heaven_acc : Outport
  tag scope: PINV_W_sp=global, PINV_Z_sp=global
  wires:
  z/1 -> Altitude Signal conditioning/1(z_In)
  vz/1 -> Unary Minus/1  "vz"
  Sum3/1 -> PID_vz/1  "vertical velocity_error"
  PID_Altitude/1 -> Gain1/1, Sum3/1  "vz_cmd"
  Altitude Signal conditioning/1(z) -> Sum2/2  "alt"
  Sum2/1 -> PID_Altitude/1
  PID_vz/1 -> heaven_acc/1  "heaven_acc"
  des_alt/1 -> Gain/1, Sum2/1  "des_alt"
  Unary Minus/1 -> Sum3/2
  Gain/1 -> [PINV_Z_sp]
  Gain1/1 -> [PINV_W_sp]
